simulink model "VehCtrlMdel241025_2018b_amkspdlimit"  (R2019b)
settings: Solver=FixedStepDiscrete  StartTime=0.0  StopTime=30  FixedStep=0.0005  RelTol=1e-3  EnableMultiTasking=on
values from neighbouring files (symbols this model uses):
  Ldwf = 0.4    [VxSpdEstiPara.m]
  Ldwr = 0.5    [VxSpdEstiPara.m]
  thr1 = 0.5    [VxSpdEstiPara.m]
  thr2 = 0.5    [VxSpdEstiPara.m]
  thr3 = 0.5    [VxSpdEstiPara.m]
  thr4 = 0.5    [VxSpdEstiPara.m]
  TrqRquRate = 20    [VxSpdEstiPara.m]
undefined symbols (not defined in the file or in its folder): Ax_OffSet, Ay_OffSet, Caf, Car, DiscIntNeverNeededParam, dwf, dwr, h, i1, i2, I_AN06_5V, I_AN07_5V, I_AN08_5V, I_AN09_5V, I_AN10_5V, I_SW01_L, I_SW02_L, I_SW03_L, I_SW05_L, I_SW07_L, Iz, Kc, Ki, Kp, lf, lr, m, O_SW01_LS0A4, O_SW02_LS0A4, O_SW04_LS0A4, O_SW05_LS0A4, O_SW06_LS0A4, O_SW07_LS0A4, O_SW08_LS0A4, O_SW09_LS0A4, O_SW12_HS1A, O_SW13_HS1A, O_SW14_HS1A, O_SW15_HS1A, Offset_Angle, PWM3, Qa, Ra, RearRatio, Rt, thr5, YawRate_OffSet
libraries: simulink x159, ec5744lib x142, canmsglib x18, MyDesignedModel x1
(part 4 of 6)

== system VehCtrlMdel241025_2018b_amkspdlimit/Input_Processing/Function-Call Subsystem/SWAS ==
  SWAS : Inport
  1-D Lookup Table : Lookup_n-D  NumberOfTableDimensions=1  BreakpointsForDimension1=|  Table=|  InternalRulePriority=Speed  RndMeth=Simplest  InputSameDT=on
      BreakpointsForDimension1=|
      | single([-119.993
      | -109.997
      | -100
      | -90.0034
      | -80.0067
      | -69.9933
      | -59.9966
      | -50
      | -40.0034
      | -30.0067
      | -19.9933
      | -9.99664
      | 0
      | 9.99664
      | 19.9933
      | 30.0067
      | 40.0034
      | 50
      | 59.9966
      | 69.9933
      | 80.0067
      | 90.0034
      | 100
      | 109.997
      | ]);
      Table=|
      | single([-26.072928
      | -23.62248
      | -20.834568
      | -18.002448
      | -15.197904
      | -12.620232
      | -10.131048
      | -8.139672
      | -6.2976672
      | -4.605012
      | -3.0893688
      | -1.4907528
      | -0.07467624
      | 1.40778
      | 2.9621448
      | 4.7211768
      | 6.5521152
      | 8.737056
      | 10.944144
      | 13.743144
      | 17.25012
      | 20.375424
      | 24.070536
      | 27.505584
      | ]);
  1-D Lookup Table1 : Lookup_n-D  NumberOfTableDimensions=1  BreakpointsForDimension1=|  Table=|  InternalRulePriority=Speed  RndMeth=Simplest  InputSameDT=on
      BreakpointsForDimension1=|
      | single([-119.995
      | -109.993
      | -99.9916
      | -90.0067
      | -80.005
      | -70.0034
      | -60.0017
      | -50
      | -39.9983
      | -29.9966
      | -19.995
      | -9.99328
      | 0.00840477
      | 9.99328
      | 19.995
      | 29.9966
      | 39.9983
      | 50
      | 60.0017
      | 70.0034
      | 80.005
      | 90.0067
      | 100.008
      | 109.993
      | ]);
      Table=|
      | single([-26.816256
      | -23.524848
      | -19.851048
      | -16.282584
      | -13.40676
      | -10.314792
      | -7.65504
      | -5.3554968
      | -3.4548912
      | -1.5044184
      | 0.02493504
      | 1.4379192
      | 2.8675296
      | 4.2638976
      | 5.76
      | 7.35588
      | 9.101304
      | 11.04624
      | 12.94128
      | 15.35724
      | 18.244152
      | 20.937168
      | 23.630112
      | 26.306496
      | ]);
  Abs : Abs
  Add1 : Sum
  Add2 : Sum
  Bus Selector : BusSelector  OutputSignals=StrWhlAng,StrWhlAngV
  Bus Creator : BusCreator  Inputs=5
  Cast To Boolean : DataTypeConversion  OutDataTypeStr=single
  Cast To Boolean1 : DataTypeConversion  OutDataTypeStr=single
  Compare To Constant : simulink/Logic and Bit Operations/Compare To Constant  relop=>  const=120  OutDataTypeStr=boolean
  Constant1 : Constant  Value=single(1200)
  Constant2 : Constant  Value=single(1200)
  Constant3 : Constant  Value=single(-1200)
  Constant4 : Constant  Value=single(-1200)
  Constant5 : Constant  Value=single(0.11)
  Gain : Gain  Gain=0.7
  Gain1 : Gain  Gain=0.3
  Gain2 : Gain  Gain=0.7
  Gain3 : Gain  Gain=0.3
  NOT : Logic  Operator=NOT  AllPortsSameDT=off  OutDataTypeStr=boolean
  Rate Limiter Dynamic : simulink/Discontinuities/Rate Limiter Dynamic
      settings: SourceProductName=Simulink
  Rate Limiter Dynamic1 : simulink/Discontinuities/Rate Limiter Dynamic
      settings: SourceProductName=Simulink
  Saturation1 : Saturate  UpperLimit=1200  LowerLimit=0
  Timer : Stateflow chart  TreatAsAtomicUnit=on
  Unit Delay : UnitDelay  SampleTime=-1  HasFrameUpgradeWarning=on
  Unit Delay1 : UnitDelay  SampleTime=-1  HasFrameUpgradeWarning=on
  StrWhlAng&V : Outport  VectorParamsAs1DForOutWhenUnconnected=off
  wires:
  SWAS/1 -> Bus Selector/1
  Bus Selector/2 -> Cast To Boolean1/1  "<StrWhlAngV>"
  Constant3/1 -> Rate Limiter Dynamic/3
  Constant2/1 -> Rate Limiter Dynamic/1
  Gain/1 -> Add2/1
  Gain1/1 -> Add2/2
  Rate Limiter Dynamic/1 -> Abs/1, Gain/1, Unit Delay/1
  Unit Delay/1 -> Gain1/1
  Add2/1 -> 1-D Lookup Table1/1, Bus Creator/4, 1-D Lookup Table/1  "StrWhlAng"
  Bus Creator/1 -> StrWhlAng&V/1
  Add1/1 -> Bus Creator/5  "StrWhlAngV"
  Rate Limiter Dynamic1/1 -> Saturation1/1
  Bus Selector/1 -> Cast To Boolean/1  "<StrWhlAng>"
  Constant1/1 -> Rate Limiter Dynamic1/1
  Constant4/1 -> Rate Limiter Dynamic1/3
  1-D Lookup Table/1 -> Bus Creator/2  "FLWhlStrAng"
  1-D Lookup Table1/1 -> Bus Creator/3  "FRWhlStrAng"
  Unit Delay1/1 -> Gain3/1
  Gain3/1 -> Add1/2
  Gain2/1 -> Add1/1
  Saturation1/1 -> Unit Delay1/1, Gain2/1  "StrWhlAngV"
  Abs/1 -> Compare To Constant/1
  NOT/1 -> Bus Creator/1  "WhlStrAng_Valid"
  Constant5/1 -> Timer/2(CountTime)
  Compare To Constant/1 -> Timer/1(Trigger)  "WhlStrAng_Valid"
  Timer/1(Exit) -> NOT/1
  Cast To Boolean/1 -> Rate Limiter Dynamic/2
  Cast To Boolean1/1 -> Rate Limiter Dynamic1/2

== system VehCtrlMdel241025_2018b_amkspdlimit/Input_Processing/Function-Call Subsystem/Subsystem ==
  note: AMK电机功率计算
  In1 : Inport
  In2 : Inport  Port=2
  In3 : Inport  Port=3
  Bus Selector : BusSelector  OutputSignals=MCFL_ActualTorque,MCFL_ActualVelocity,MCFL_DCVoltage
  Bus Selector1 : BusSelector  OutputSignals=MCFR_ActualTorque,MCFR_ActualVelocity,MCFR_DCVoltage
  Bus Selector2 : BusSelector  OutputSignals=voltage,current
  Constant : Constant  Value=single(9550)
  Constant1 : Constant  Value=single(9550)
  Constant2 : Constant  Value=single(0.01)
  Constant3 : Constant  Value=single(0.01)
  Constant4 : Constant  Value=single(0)
  Constant6 : Constant  Value=single(0)
  Divide{,1..3} (4 alike) : Product  Inputs=*/
  Max : MinMax  Function=max  Inputs=2
  Max1 : MinMax  Function=max  Inputs=2
  MeaModule : ec5744lib/RapidECU_U3/07Calibration/MeaModule  signal=AMKFL_Current
      settings: SourceProductName=ECUCoder for MPC5744
  MeaModule1 : ec5744lib/RapidECU_U3/07Calibration/MeaModule  signal=AMKFR_Current
      settings: SourceProductName=ECUCoder for MPC5744
  MeaModule2 : ec5744lib/RapidECU_U3/07Calibration/MeaModule  signal=EmraxPwr
      settings: SourceProductName=ECUCoder for MPC5744
  Product : Product
  Product1 : Product
  Product2 : Product
  Switch : Switch  Criteria=u2 ~= 0
  Switch1 : Switch  Criteria=u2 ~= 0
  Out1 : Outport
  Out2 : Outport  Port=2
  Out3 : Outport  Port=3
  wires:
  In1/1 -> Bus Selector/1
  In2/1 -> Bus Selector1/1
  Bus Selector/1 -> Product/1  "<MCFL_ActualTorque>"
  Bus Selector/2 -> Product/2  "<MCFL_ActualVelocity>"
  Bus Selector/3 -> Switch/2, Max/1  "<MCFL_DCVoltage>"
  Product/1 -> Divide/1
  Constant/1 -> Divide/2
  Switch/1 -> MeaModule/1  "AMKFL_Current"
  Constant1/1 -> Divide2/2
  Product1/1 -> Divide2/1
  Bus Selector1/3 -> Switch1/2, Max1/1  "<MCFR_DCVoltage>"
  Bus Selector1/1 -> Product1/1  "<MCFR_ActualTorque>"
  Bus Selector1/2 -> Product1/2  "<MCFR_ActualVelocity>"
  Switch1/1 -> MeaModule1/1  "AMKFR_Current"
  MeaModule/1 -> Out1/1
  MeaModule1/1 -> Out2/1
  Constant2/1 -> Max/2
  Max/1 -> Divide1/2
  Constant3/1 -> Max1/2
  Max1/1 -> Divide3/2
  Divide1/1 -> Switch/1  "AMKFL_Current"
  Constant4/1 -> Switch/3
  Constant6/1 -> Switch1/3
  Divide3/1 -> Switch1/1  "AMKFR_Current"
  In3/1 -> Bus Selector2/1
  Bus Selector2/2 -> Product2/2  "<current>"
  Bus Selector2/1 -> Product2/1  "<voltage>"
  Product2/1 -> MeaModule2/1
  MeaModule2/1 -> Out3/1
  Divide/1 -> Divide1/1
  Divide2/1 -> Divide3/1

== system VehCtrlMdel241025_2018b_amkspdlimit/Input_Processing/Function-Call Subsystem/Subsystem1 ==
  In1 : Inport
  Bus Selector : BusSelector  OutputSignals=FLAMKMCUtoVCU1.MCFL_bError,FRAMKMCUtoVCU1.MCFR_bError
  Chart : Stateflow chart  BlockKeywords=__PRM__SERIALIZED__DATA__:Stateflow Chart,Stateflow Diagram  TreatAsAtomicUnit=on
  Constant1 : Constant  Value=single(0.2)
  Detect Rise Positive1 : simulink/Logic and Bit Operations/Detect Rise Positive  vinit=0  OutDataTypeStr=boolean
  OR : Logic  Operator=OR  AllPortsSameDT=off  OutDataTypeStr=boolean
  Timer : Stateflow chart  TreatAsAtomicUnit=on
  AMKerrorTrq_CUT : Outport
  wires:
  In1/1 -> Bus Selector/1
  Bus Selector/1 -> OR/1  "<MCFL_bError>"
  Bus Selector/2 -> OR/2  "<MCFR_bError>"
  OR/1 -> Timer/1(Trigger)
  Constant1/1 -> Timer/2(CountTime)
  Timer/1(Exit) -> Detect Rise Positive1/1
  Detect Rise Positive1/1 -> Chart/1(out1)  "out1"
  Chart/1(Trq_CUT) -> AMKerrorTrq_CUT/1

== system VehCtrlMdel241025_2018b_amkspdlimit/Input_Processing/Function-Call Subsystem/WhlSpdii_mps ==
  IMU : Inport
  In2 : Inport  Port=2
  Bus Selector : BusSelector  OutputSignals=ABS_WS_RL,ABS_WS_RR
  Bus Selector1 : BusSelector  OutputSignals=FRAMKMCUtoVCU1.MCFR_ActualVelocity,FLAMKMCUtoVCU1.MCFL_ActualVelocity
  Bus Creator : BusCreator  Inputs=8
  Compare To Constant{,2,4,6} (4 alike) : simulink/Logic and Bit Operations/Compare To Constant  relop=>=  const=0  OutDataTypeStr=boolean
  Compare To Constant{1,3,5,7} (4 alike) : simulink/Logic and Bit Operations/Compare To Constant  relop=<  const=40  OutDataTypeStr=boolean
  Constant{1,4..5,8} (4 alike) : Constant  Value=single(0.11)
  Constant{2,6,10,12} (4 alike) : Constant  Value=single(10)
  Constant{3,7,11,13} (4 alike) : Constant  Value=single(-10)
  Gain : Gain  Gain=1/3.6
  Gain1 : Gain  Gain=0.4826*3.14/11.3/60
  Gain2 : Gain  Gain=0.4826*3.14/11.3/60
  Gain3 : Gain  Gain=1/3.6
  OR{,1..3} (4 alike) : Logic  Operator=OR  AllPortsSameDT=off  OutDataTypeStr=boolean
  Rate Limiter Dynamic{,1..3} (4 alike) : simulink/Discontinuities/Rate Limiter Dynamic
      settings: SourceProductName=Simulink
  Saturation{,1..3} (4 alike) : Saturate  UpperLimit=30  LowerLimit=0
  Timer : Stateflow chart  TreatAsAtomicUnit=on
  Timer1 : Stateflow chart  TreatAsAtomicUnit=on
  Timer2 : Stateflow chart  TreatAsAtomicUnit=on
  Timer3 : Stateflow chart  TreatAsAtomicUnit=on
  WhlSpdii_mps : Outport  VectorParamsAs1DForOutWhenUnconnected=off
  wires:
  IMU/1 -> Bus Selector/1
  Bus Selector/1 -> Rate Limiter Dynamic/2  "<ABS_WS_RL>"
  Bus Selector/2 -> Rate Limiter Dynamic1/2  "<ABS_WS_RR>"
  Constant2/1 -> Rate Limiter Dynamic/1
  Constant3/1 -> Rate Limiter Dynamic/3
  Constant7/1 -> Rate Limiter Dynamic1/3
  Constant6/1 -> Rate Limiter Dynamic1/1
  Constant10/1 -> Rate Limiter Dynamic2/1
  Constant11/1 -> Rate Limiter Dynamic2/3
  Bus Selector1/1 -> Rate Limiter Dynamic2/2  "<MCFR_ActualVelocity>"
  Bus Selector1/2 -> Rate Limiter Dynamic3/2  "<MCFL_ActualVelocity>"
  Constant13/1 -> Rate Limiter Dynamic3/3
  Constant12/1 -> Rate Limiter Dynamic3/1
  In2/1 -> Bus Selector1/1
  Rate Limiter Dynamic/1 -> Saturation/1
  Rate Limiter Dynamic1/1 -> Saturation1/1
  Rate Limiter Dynamic2/1 -> Saturation2/1
  Rate Limiter Dynamic3/1 -> Saturation3/1
  Saturation/1 -> Gain/1  "WhlSpdRL"
  Saturation1/1 -> Gain3/1  "WhlSpdRR"
  Saturation2/1 -> Gain1/1  "WhlSpdFR"
  Saturation3/1 -> Gain2/1  "WhlSpdFL"
  Bus Creator/1 -> WhlSpdii_mps/1
  Gain2/1 -> Compare To Constant6/1, Compare To Constant7/1, Bus Creator/8  "WhlSpdFL"
  Gain1/1 -> Compare To Constant5/1, Compare To Constant4/1, Bus Creator/6  "WhlSpdFR"
  Gain/1 -> Compare To Constant/1, Compare To Constant1/1, Bus Creator/2  "WhlSpdRL_mps"
  Gain3/1 -> Compare To Constant2/1, Compare To Constant3/1, Bus Creator/4  "WhlSpdRR_mps"
  Compare To Constant/1 -> OR/1
  Compare To Constant1/1 -> OR/2
  Compare To Constant3/1 -> OR1/2
  Compare To Constant2/1 -> OR1/1
  Compare To Constant4/1 -> OR2/1
  Compare To Constant5/1 -> OR2/2
  Compare To Constant7/1 -> OR3/2
  Compare To Constant6/1 -> OR3/1
  Timer/1(Exit) -> Bus Creator/1  "WhlSpdRL_Valid"
  Timer1/1(Exit) -> Bus Creator/3  "WhlSpdRR_Valid"
  Timer2/1(Exit) -> Bus Creator/5  "WhlSpdFR_Valid"
  Timer3/1(Exit) -> Bus Creator/7  "WhlSpdFL_Valid"
  Constant5/1 -> Timer/2(CountTime)
  OR/1 -> Timer/1(Trigger)  "WhlSpdRL_Valid"
  OR1/1 -> Timer1/1(Trigger)  "WhlSpdRR_Valid"
  Constant1/1 -> Timer1/2(CountTime)
  Constant4/1 -> Timer2/2(CountTime)
  OR2/1 -> Timer2/1(Trigger)  "WhlSpdFR_Valid"
  Constant8/1 -> Timer3/2(CountTime)
  OR3/1 -> Timer3/1(Trigger)  "WhlSpdFL_Valid"

== system VehCtrlMdel241025_2018b_amkspdlimit/Input_Processing/Subsystem/IntglJudgment  ==
  note: 对加速度进行积分
  note: 计时器，当积分速度大于轮速一个时间后，退出积分速度。
  note: 积分开始时，需要给初始值
  WhlSlipFL_flag : Inport
  WhlSlipFR_flag : Inport  Port=2
  WhlSlipRL_flag : Inport  Port=3
  WhlSlipRR_flag : Inport  Port=4
  Ax_Valid : Inport  Port=5
  IMU_Ax_mpss : Inport  Port=6
  FFVehVxEst_mps : Inport  Port=7
  Acc_POS : Inport  Port=8
  WhlSpdMax_mps : Inport  Port=9
  AND : Logic  AllPortsSameDT=off  OutDataTypeStr=boolean
  Add{,3..4,10} (4 alike) : Sum
  Add1 : Sum  Inputs=-+
  Add2 : Sum  Inputs=+-
  Cast To Double : DataTypeConversion  OutDataTypeStr=single
  Cast To Double1 : DataTypeConversion  OutDataTypeStr=boolean
  Compare To Constant : simulink/Logic and Bit Operations/Compare To Constant  relop=>  const=TrqRquRate  OutDataTypeStr=boolean
  Compare To Constant1 : simulink/Logic and Bit Operations/Compare To Constant  relop=<=  const=0  OutDataTypeStr=boolean
  Constant : Constant  Value=single(0)
  InitZORE : Constant  Value=single(0)
  Logical Operator : Logic  Operator=OR  Inputs=4  AllPortsSameDT=off  OutDataTypeStr=boolean
  Logical Operator1 : Logic  Operator=NOT  AllPortsSameDT=off  OutDataTypeStr=boolean
  Logical Operator2 : Logic  Operator=OR  AllPortsSameDT=off  OutDataTypeStr=boolean
  Logical Operator3 : Logic  Operator=NOT  AllPortsSameDT=off  OutDataTypeStr=boolean
  Min : MinMax  Inputs=2
  Product : Product
  Relational Operator9 : RelationalOperator  OutDataTypeStr=boolean  RndMeth=Simplest
  Reset : Constant  Value=single(0)
  ResetDelay : Constant  Value=single(0.1)
  Saturation : Saturate  UpperLimit=200  LowerLimit=-10
  Saturation1 : Saturate  UpperLimit=200  LowerLimit=-10
  Steptime : Constant  Value=single(0.01)
  Switch{1,3..4,6} (4 alike) : Switch  Criteria=u2 ~= 0
  Unit Delay{,1..4} (5 alike) : UnitDelay  SampleTime=-1  HasFrameUpgradeWarning=on
  steptime1 : Constant  Value=single(0.01)
  steptime2 : Constant  Value=single(0)
  VxIMU_est : Outport
  IMUVehSpdEstiExit : Outport  Port=2
  wires:
  WhlSlipFL_flag/1 -> Logical Operator/1
  WhlSlipFR_flag/1 -> Logical Operator/2
  WhlSlipRL_flag/1 -> Logical Operator/3
  WhlSlipRR_flag/1 -> Logical Operator/4
  Logical Operator/1 -> Logical Operator1/1
  Unit Delay/1 -> Saturation1/1
  Add/1 -> Switch1/1
  Constant/1 -> Switch1/3
  Logical Operator1/1 -> Logical Operator2/1
  Acc_POS/1 -> Cast To Double/1
  Unit Delay4/1 -> Add1/1
  Add1/1 -> Compare To Constant/1
  Compare To Constant/1 -> Logical Operator2/2
  [IMUAccIns_ACT] -> Switch1/2
  Logical Operator2/1 -> Cast To Double1/1
  Add2/1 -> Compare To Constant1/1
  WhlSpdMax_mps/1 -> Add2/1
  Saturation1/1 -> Add/2
  Product/1 -> Add/1
  IMU_Ax_mpss/1 -> Product/1
  steptime1/1 -> Product/2
  Saturation/1 -> Add3/1
  Add3/1 -> Add2/2, VxIMU_est/1  "VxIMU_est"
  Switch6/1 -> Min/1
  ResetDelay/1 -> Relational Operator9/2, Min/2
  Compare To Constant1/1 -> Switch6/2
  Add10/1 -> Switch6/1
  Steptime/1 -> Add10/2
  Min/1 -> Relational Operator9/1, Unit Delay2/1
  Reset/1 -> Switch6/3
  Unit Delay2/1 -> Add10/1
  Unit Delay3/1 -> Logical Operator3/1
  InitZORE/1 -> Switch4/3
  Logical Operator3/1 -> Switch3/2
  Switch3/1 -> Add3/2, Unit Delay1/1  "VehSpdInit_mps"
  Switch4/1 -> Switch3/1
  Cast To Double/1 -> Unit Delay4/1, Add1/2
  [IMUAccIns_ACT] -> Unit Delay3/1, Switch4/2  "IMUAccIns_ACT"
  Relational Operator9/1 -> IMUVehSpdEstiExit/1  "IMUVehSpdEstiExit"
  Cast To Double1/1 -> AND/2
  Unit Delay1/1 -> Switch3/3
  Add4/1 -> Switch4/1
  FFVehVxEst_mps/1 -> Add4/2
  steptime2/1 -> Add4/1
  Switch1/1 -> Saturation/1, Unit Delay/1
  AND/1 -> [IMUAccIns_ACT]
  Ax_Valid/1 -> AND/1

== system VehCtrlMdel241025_2018b_amkspdlimit/Input_Processing/Subsystem/WhlSlpageJudgment ==
  note: 实践中很难同时满足这三个条件。
      | 一般只满足后两个其中一个即可。
  note: 更改记录：1、理了信号线，更整齐。
      | 2、加速度差，加速度差的微分的判断加入滤波模块。
      | 3、轮速选取改为选取最大轮速。
  note: 选取一个最大轮速
  Vxii_mps : Inport
  IMU_YawRate_dps : Inport  Port=2
  IMU_Aa_mpss : Inport  Port=3
  VehSpdEstiZ1_mps : Inport  Port=4
  In5 : Inport  Port=5
  Bus Selector : BusSelector  OutputSignals=VxFL_mps,VxFR_mps,VxRL_mps,VxRR_mps
  Cast To Double{,1..3} (4 alike) : DataTypeConversion  OutDataTypeStr=boolean
  Constant{1..4} (4 alike) : Constant  Value=single(0.5)
  Logical Operator : Logic  Operator=OR  AllPortsSameDT=off  OutDataTypeStr=boolean
  Logical Operator1 : Logic  AllPortsSameDT=off  OutDataTypeStr=boolean
  Min1 : MinMax  Function=max  Inputs=4
  Mux : Mux
  Mux1 : Mux
  Mux2 : Mux
  Selector : Selector  InputPortWidth=4  IndexOptions=Index vector (dialog)  Indices=[1]  OutputSizes=1
  Selector1 : Selector  InputPortWidth=4  IndexOptions=Index vector (dialog)  Indices=[2]  OutputSizes=1
  Selector2 : Selector  InputPortWidth=4  IndexOptions=Index vector (dialog)  Indices=[3]  OutputSizes=1
  Selector3 : Selector  InputPortWidth=4  IndexOptions=Index vector (dialog)  Indices=[4]  OutputSizes=1
  Terminator : Terminator
  Timer : Stateflow chart  TreatAsAtomicUnit=on
  Timer1 : Stateflow chart  TreatAsAtomicUnit=on
  Timer2 : Stateflow chart  TreatAsAtomicUnit=on
  Timer3 : Stateflow chart  TreatAsAtomicUnit=on
  加速度差判断 : Subsystem
  加速度差的微分的判断 : Subsystem
  速差判断 : Subsystem
  WhlSlipFLValid_flag : Outport
  WhlSlipFRValid_flag : Outport  Port=2
  WhlSlipRLValid_flag : Outport  Port=3
  WhlSlipRRValid_flag : Outport  Port=4
  WhlSpdMax_mps : Outport  Port=5
  wires:
  Selector3/1 -> Cast To Double3/1
  Selector2/1 -> Cast To Double2/1
  [IMU_Aa_mpsss] -> 加速度差的微分的判断/5(IMU_Ax_mpss)
  [VehSpdEstiZ1_mps] -> 速差判断/5(VehSpd_mps)
  Bus Selector/3 -> 加速度差的微分的判断/3(<VxRL_mps>), Min1/3, 速差判断/3(<VxRL_mps>), 加速度差判断/3(<VxRL_mps>)  "<VxRL_mps>"
  Selector1/1 -> Cast To Double1/1
  [IMU_Aa_mpsss] -> 加速度差判断/5(IMU_Ax_mpss)
  Bus Selector/4 -> 加速度差判断/4(<VxRR_mps>), Min1/4, 速差判断/4(<VxRR_mps>), 加速度差的微分的判断/4(<VxRR_mps>)  "<VxRR_mps>"
  IMU_YawRate_dps/1 -> [IMU_YawRate_dps]
  Vxii_mps/1 -> Bus Selector/1
  Bus Selector/1 -> 加速度差的微分的判断/1(<VxFL_mps>), 加速度差判断/1(<VxFL_mps>), Min1/1, 速差判断/1(<VxFL_mps>)  "<VxFL_mps>"
  VehSpdEstiZ1_mps/1 -> [VehSpdEstiZ1_mps]
  Selector/1 -> Cast To Double/1
  Bus Selector/2 -> 加速度差的微分的判断/2(<VxFR_mps>), 加速度差判断/2(<VxFR_mps>), Min1/2, 速差判断/2(<VxFR_mps>)  "<VxFR_mps>"
  IMU_Aa_mpss/1 -> [IMU_Aa_mpsss]
  [IMU_YawRate_dps] -> Terminator/1
  Timer/1(Exit) -> WhlSlipFLValid_flag/1  "WhlSlipFLValid_flag"
  Cast To Double2/1 -> Timer2/1(Trigger)  "WhlSlipRLValid_flag"
  Cast To Double3/1 -> Timer3/1(Trigger)  "WhlSlipRRValid_flag"
  速差判断/1(y) -> Mux/1  "速差"
  速差判断/2(y1) -> Mux/2
  速差判断/3(y2) -> Mux/3
  速差判断/4(y3) -> Mux/4
  加速度差判断/1(y) -> Mux1/1  "加速度差"
  加速度差判断/2(y1) -> Mux1/2
  加速度差判断/3(y2) -> Mux1/3
  加速度差判断/4(y3) -> Mux1/4
  加速度差的微分的判断/1(y) -> Mux2/1  "加速度差的微分"
  加速度差的微分的判断/2(y1) -> Mux2/2
  加速度差的微分的判断/3(y2) -> Mux2/3
  加速度差的微分的判断/4(y3) -> Mux2/4
  Mux1/1 -> Logical Operator/1
  Mux2/1 -> Logical Operator/2
  Mux/1 -> Logical Operator1/1
  Logical Operator/1 -> Logical Operator1/2
  Logical Operator1/1 -> Selector3/1, Selector2/1, Selector1/1, Selector/1
  Min1/1 -> WhlSpdMax_mps/1
  In5/1 -> 速差判断/6(In6)
  Constant1/1 -> Timer/2(CountTime)
  Cast To Double/1 -> Timer/1(Trigger)  "WhlSlipFLValid_flag"
  Timer1/1(Exit) -> WhlSlipFRValid_flag/1  "WhlSlipFRValid_flag"
  Cast To Double1/1 -> Timer1/1(Trigger)  "WhlSlipFRValid_flag"
  Timer2/1(Exit) -> WhlSlipRLValid_flag/1  "WhlSlipRLValid_flag"
  Timer3/1(Exit) -> WhlSlipRRValid_flag/1  "WhlSlipRRValid_flag"
  Constant2/1 -> Timer1/2(CountTime)
  Constant3/1 -> Timer2/2(CountTime)
  Constant4/1 -> Timer3/2(CountTime)

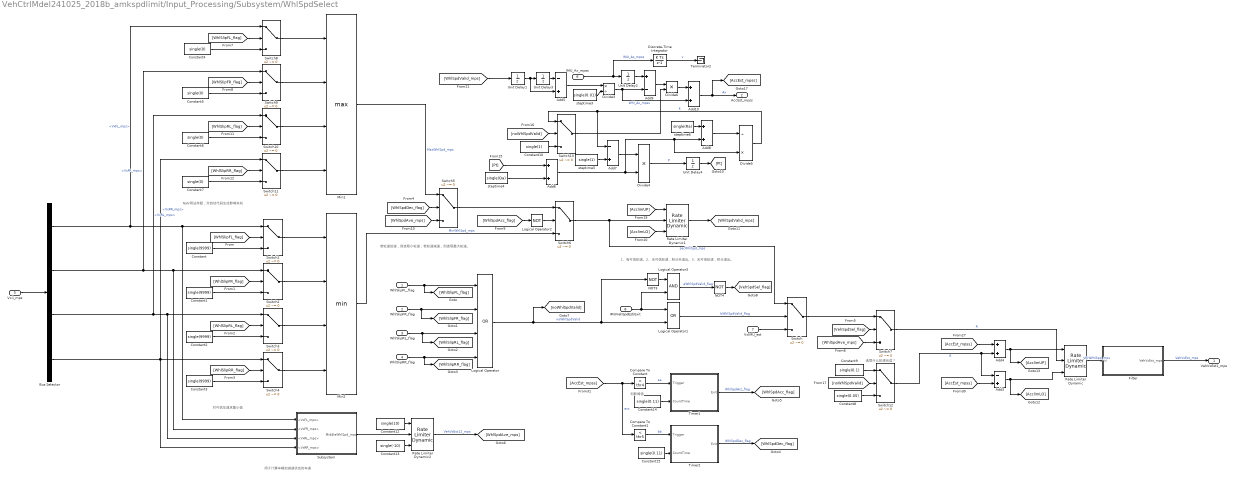
== system VehCtrlMdel241025_2018b_amkspdlimit/Input_Processing/Subsystem/WhlSpdSelect ==
  note: 用于计算车辆加减速状态的车速
  note: 1、有可信轮速。2、无可信轮速，积分未退出。3、无可信轮速，积分退出。
  note: 选取什么轮速合适？
  note: 判断阈值
  note: 若轮速加速，则选取小轮速；若轮速减速，则选取最大轮速。
  note: NaN用法存疑，对自动代码生成影响未知
  note: 对可信车速求最小值
  WhlSlipFL_flag : Inport
  WhlSlipFR_flag : Inport  Port=2
  WhlSlipRL_flag : Inport  Port=3
  WhlSlipRR_flag : Inport  Port=4
  Vxii_mps : Inport  Port=5
  IMU_Ax_mpss : Inport  Port=6
  VxIMU_est : Inport  Port=7
  IMUVehSpdEstiExit : Inport  Port=8
  Add{4,6,8,10} (4 alike) : Sum
  Add3 : Sum  Inputs=-+
  Add5 : Sum  Inputs=-+
  Add7 : Sum  Inputs=-+
  Add9 : Sum  Inputs=+-
  Bus Selector : BusSelector  OutputSignals=VxFL_mps,VxFR_mps,VxRL_mps,VxRR_mps
  Compare To Constant : simulink/Logic and Bit Operations/Compare To Constant  relop=>  const=thr4  OutDataTypeStr=boolean
  Compare To Constant1 : simulink/Logic and Bit Operations/Compare To Constant  relop=<  const=thr5  OutDataTypeStr=boolean
  Constant{,1..3} (4 alike) : Constant  Value=single(9999)
  Constant10 : Constant  Value=single(1)
  Constant12 : Constant  Value=single(10)
  Constant13 : Constant  Value=single(-10)
  Constant14 : Constant  Value=single(0.11)
  Constant15 : Constant  Value=single(0.11)
  Constant{4..7} (4 alike) : Constant  Value=single(0)
  Constant8 : Constant  Value=single(0.05)
  Constant9 : Constant  Value=single(0.1)
  Discrete-Time Integrator : DiscreteIntegrator  SampleTime=-1  ICPrevOutput=DiscIntNeverNeededParam  ICPrevScaledInput=DiscIntNeverNeededParam
  Divide3 : Product  Inputs=*/
  Divide4 : Product  Inputs=**
  Divide5 : Product  Inputs=/*
  Divide6 : Product  Inputs=**
  Filter : Subsystem
  Logical Operator : Logic  Operator=OR  Inputs=4  AllPortsSameDT=off  OutDataTypeStr=boolean
  Logical Operator1 : Logic  Operator=OR  AllPortsSameDT=off  OutDataTypeStr=boolean
  Logical Operator2 : Logic  Operator=NOT  AllPortsSameDT=off  OutDataTypeStr=boolean
  Logical Operator3 : Logic  AllPortsSameDT=off  OutDataTypeStr=boolean
  Min1 : MinMax  Function=max  Inputs=4
  Min2 : MinMax  Inputs=4
  NOT3 : Logic  Operator=NOT  AllPortsSameDT=off  OutDataTypeStr=boolean
  NOT4 : Logic  Operator=NOT  AllPortsSameDT=off  OutDataTypeStr=boolean
  Rate Limiter Dynamic : simulink/Discontinuities/Rate Limiter Dynamic
      settings: SourceProductName=Simulink
  Rate Limiter Dynamic1 : simulink/Discontinuities/Rate Limiter Dynamic
      settings: SourceProductName=Simulink
  Rate Limiter Dynamic2 : simulink/Discontinuities/Rate Limiter Dynamic
      settings: SourceProductName=Simulink
  Subsystem : Subsystem
  Switch{,1..13} (14 alike) : Switch  Criteria=u2 ~= 0
  Terminator2 : Terminator
  Timer1 : Stateflow chart  TreatAsAtomicUnit=on
  Timer2 : Stateflow chart  TreatAsAtomicUnit=on
  Unit Delay1 : UnitDelay  SampleTime=-1  HasFrameUpgradeWarning=on
  Unit Delay2 : UnitDelay  SampleTime=-1  HasFrameUpgradeWarning=on
  Unit Delay3 : UnitDelay  SampleTime=-1  HasFrameUpgradeWarning=on
  Unit Delay4 : UnitDelay  InitialCondition=0.01  SampleTime=-1  HasFrameUpgradeWarning=on
  steptime3 : Constant  Value=single(0.01)
  steptime4 : Constant  Value=single(Qa)
  steptime5 : Constant  Value=single(1)
  steptime6 : Constant  Value=single(Ra)
  VehVxEst1_mps : Outport
  AccEst_mpss : Outport  Port=2
  wires:
  Compare To Constant/1 -> Timer1/1(Trigger)  "aa"
  Vxii_mps/1 -> Bus Selector/1
  WhlSlipRR_flag/1 -> [WhlSlipRR_flag], Logical Operator/4
  Logical Operator3/1 -> NOT4/1  "aWhlSpdValid_flag"
  [VehSpdSel_flag] -> Switch7/2
  Logical Operator2/1 -> Switch6/2
  [WhlSlipFL_flag] -> Switch1/2
  Switch5/1 -> Switch6/1
  Constant/1 -> Switch1/3
  Compare To Constant1/1 -> Timer2/1(Trigger)  "bb"
  [WhlSpdAve_mps] -> Switch5/3
  Constant3/1 -> Switch4/3
  Logical Operator1/1 -> Switch/2  "bWhlSpdValid_flag"
  Switch4/1 -> Min2/4
  Constant2/1 -> Switch3/3
  [WhlSlipRR_flag] -> Switch4/2
  Switch1/1 -> Min2/1
  WhlSlipFR_flag/1 -> [WhlSlipFR_flag], Logical Operator/2
  [WhlSpdAcc_flag] -> Logical Operator2/1
  [WhlSlipRL_flag] -> Switch3/2
  Switch2/1 -> Min2/2
  WhlSlipFL_flag/1 -> [WhlSlipFL_flag], Logical Operator/1
  Constant1/1 -> Switch2/3
  [WhlSpdDec_flag] -> Switch5/2
  [WhlSlipFR_flag] -> Switch2/2
  WhlSlipRL_flag/1 -> [WhlSlipRL_flag], Logical Operator/3
  Switch3/1 -> Min2/3
  [WhlSpdAve_mps] -> Switch7/3
  Bus Selector/1 -> Switch8/1, Subsystem/1(<VxFL_mps>), Switch1/1  "<VxFL_mps>"
  Bus Selector/4 -> Subsystem/4(<VxRR_mps>), Switch11/1, Switch4/1  "<VxRR_mps>"
  [WhlSlipFR_flag] -> Switch9/2
  Bus Selector/2 -> Switch9/1, Subsystem/2(<VxFR_mps>), Switch2/1  "<VxFR_mps>"
  Constant5/1 -> Switch9/3
  Bus Selector/3 -> Switch10/1, Subsystem/3(<VxRL_mps>), Switch3/1  "<VxRL_mps>"
  [WhlSlipRL_flag] -> Switch10/2
  [WhlSlipRR_flag] -> Switch11/2
  Constant6/1 -> Switch10/3
  Constant7/1 -> Switch11/3
  Constant4/1 -> Switch8/3
  [WhlSlipFL_flag] -> Switch8/2
  Switch8/1 -> Min1/1
  Switch9/1 -> Min1/2
  Switch10/1 -> Min1/3
  Switch11/1 -> Min1/4
  Min1/1 -> Switch5/1  "MaxWhlSpd_mps"
  Subsystem/1(MiddleWhlSpd_mps) -> Rate Limiter Dynamic2/2
  Constant12/1 -> Rate Limiter Dynamic2/1
  Constant13/1 -> Rate Limiter Dynamic2/3
  Rate Limiter Dynamic2/1 -> [WhlSpdAve_mps]  "VehVxEst12_mps"
  Min2/1 -> Switch6/3  "MinWhlSpd_mps"
  IMUVehSpdEstiExit/1 -> Logical Operator3/2, Logical Operator1/1
  NOT3/1 -> Logical Operator3/1
  NOT4/1 -> [VehSpdSel_flag]
  Divide5/1 -> Add7/1, Switch13/1  "K"
  Unit Delay3/1 -> Add5/1
  steptime3/1 -> Divide3/2
  Add5/1 -> Divide3/1
  Unit Delay4/1 -> [Pt]
  [Pt] -> Add6/1
  steptime4/1 -> Add6/2
  Add6/1 -> Divide5/2, Add8/2, Divide4/2
  steptime5/1 -> Add7/2
  Add7/1 -> Divide4/1
  Divide4/1 -> Unit Delay4/1  "P"
  steptime6/1 -> Add8/1
  Add8/1 -> Divide5/1
  Divide3/1 -> Add10/2, Add9/2  "Whl_Ax_mpss"
  Add9/1 -> Divide6/1
  Divide6/1 -> Add10/1
  Add10/1 -> AccEst_mpss/1, [AccEst_mpss]  "Ax"
  IMU_Ax_mpss/1 -> Unit Delay2/1, Discrete-Time Integrator/1  "IMU_Ax_mpss"
  VxIMU_est/1 -> Switch/3
  Filter/1(VehVxEst_mps) -> VehVxEst1_mps/1  "VehVxEst_mps"
  Switch/1 -> Switch7/1
  Discrete-Time Integrator/1 -> Terminator2/1  "v"
  [AccEst_mpss] -> Add4/1
  [AccEst_mpss] -> Add3/2
  [WhlSpdValid_mps] -> Unit Delay1/1
  Unit Delay2/1 -> Add9/1
  Switch6/1 -> Switch/1, Rate Limiter Dynamic1/2  "secWhlSpd_mps"
  Add4/1 -> [AcclimUP], Rate Limiter Dynamic/1
  Add3/1 -> [AcclimLO], Rate Limiter Dynamic/3
  Switch7/1 -> Rate Limiter Dynamic/2  "R"
  Rate Limiter Dynamic/1 -> Filter/1(In)  "VEHWhlSpd_mps"
  Rate Limiter Dynamic1/1 -> [WhlSpdValid_mps]
  Unit Delay1/1 -> Add5/2, Unit Delay3/1
  [noWhlSpdValid] -> Switch12/2
  Constant8/1 -> Switch12/3
  Constant9/1 -> Switch12/1
  Switch12/1 -> Add3/1, Add4/2  "R"
  Switch13/1 -> Divide6/2
  [noWhlSpdValid] -> Switch13/2
  Constant10/1 -> Switch13/3
  [AcclimUP] -> Rate Limiter Dynamic1/1
  [AcclimLO] -> Rate Limiter Dynamic1/3
  Logical Operator/1 -> NOT3/1, Logical Operator1/2, [noWhlSpdValid]  "noWhlSpdValid"
  Timer1/1(Exit) -> [WhlSpdAcc_flag]  "WhlSpdAcc_flag"
  Constant14/1 -> Timer1/2(CountTime)
  Timer2/1(Exit) -> [WhlSpdDec_flag]  "WhlSpdDec_flag"
  Constant15/1 -> Timer2/2(CountTime)
  [AccEst_mpss] -> Compare To Constant1/1, Compare To Constant/1  "acc"

== system VehCtrlMdel241025_2018b_amkspdlimit/Input_Processing/Subsystem/坐标系转换 ==
  note: cos模块的单位是弧度制、
  note: 未考虑漂移工况
  note: 顺时针为正，逆时针为负。
  WhlSpdFL_mps : Inport
  WhlSpdFR_mps : Inport  Port=2
  WhlSpdRL_mps : Inport  Port=3
  WhlSpdRR_mps : Inport  Port=4
  IMU_YawRate_dps : Inport  Port=5
  WhlStrAngL_deg : Inport  Port=6
  WhlStrAngR_deg : Inport  Port=7
  Add : Sum  Inputs=+-
  Add1 : Sum
  Add2 : Sum  Inputs=+-
  Add3 : Sum
  Asin : Trigonometry  Operator=cos
  Asin1 : Trigonometry  Operator=cos
  Bus Creator : BusCreator  Inputs=4
  Constant : Constant  Value=single(Ldwr)
  Constant1 : Constant  Value=single(Ldwf)
  Gain : Gain  Gain=1/2
  Gain1 : Gain  Gain=1/2
  Gain2 : Gain  Gain=pi/180
  Gain3 : Gain  Gain=pi/180
  Gain4 : Gain  Gain=pi/180
  Product{,1..3} (4 alike) : Product
  Vxii_mps : Outport
  IMU_YawRate_dps1 : Outport  Port=2
  wires:
  Constant/1 -> Gain/1
  Gain/1 -> Product/2
  IMU_YawRate_dps/1 -> Gain4/1  "IMU_YawRate_dps"
  WhlSpdRL_mps/1 -> Add/1  "WhlSpdRL_mps"
  WhlSpdRR_mps/1 -> Add1/2  "WhlSpdRR_mps"
  Product/1 -> [Vldwr]
  [Vldwr] -> Add/2, Add1/1
  WhlSpdFL_mps/1 -> Product1/1  "WhlSpdFL_mps"
  WhlSpdFR_mps/1 -> Product2/2  "WhlSpdFR_mps"
  Constant1/1 -> Gain1/1
  Gain1/1 -> Product3/1
  Product3/1 -> [Vldwf]
  Product1/1 -> Add2/1  "1"
  [Vldwf] -> Add2/2, Add3/1  "3"
  Product2/1 -> Add3/2
  Add2/1 -> Bus Creator/1  "VxFL_mps"
  Add/1 -> Bus Creator/3  "VxRL_mps"
  Add3/1 -> Bus Creator/2  "VxFR_mps"
  Add1/1 -> Bus Creator/4  "VxRR_mps"
  Bus Creator/1 -> Vxii_mps/1
  Asin1/1 -> Product2/1
  WhlStrAngR_deg/1 -> Gain3/1  "WhlStrAngR_deg"
  WhlStrAngL_deg/1 -> Gain2/1  "WhlStrAngL_deg"
  Asin/1 -> Product1/2  "a"
  Gain2/1 -> Asin/1
  Gain3/1 -> Asin1/1
  Gain4/1 -> IMU_YawRate_dps1/1, Product/1, Product3/2

== system VehCtrlMdel241025_2018b_amkspdlimit/OUTPUT/Beeper/Enabled Subsystem1 ==
  In1 : Inport
  In2 : Inport  Port=2
  Enable : EnablePort
  Chart : Stateflow chart  BlockKeywords=__PRM__SERIALIZED__DATA__:Stateflow Chart,Stateflow Diagram  TreatAsAtomicUnit=on
  Error_State : Outport
  wires:
  In1/1 -> Chart/2(FL)
  In2/1 -> Chart/1(FR)
  Chart/1(LEDOn) -> Error_State/1

== system VehCtrlMdel241025_2018b_amkspdlimit/OUTPUT/Beeper/Subsystem ==
  Enable : EnablePort
  Chart1 : Stateflow chart  BlockKeywords=__PRM__SERIALIZED__DATA__:Stateflow Chart,Stateflow Diagram  TreatAsAtomicUnit=on
  Out1 : Outport
  wires:
  Chart1/1(led) -> Out1/1

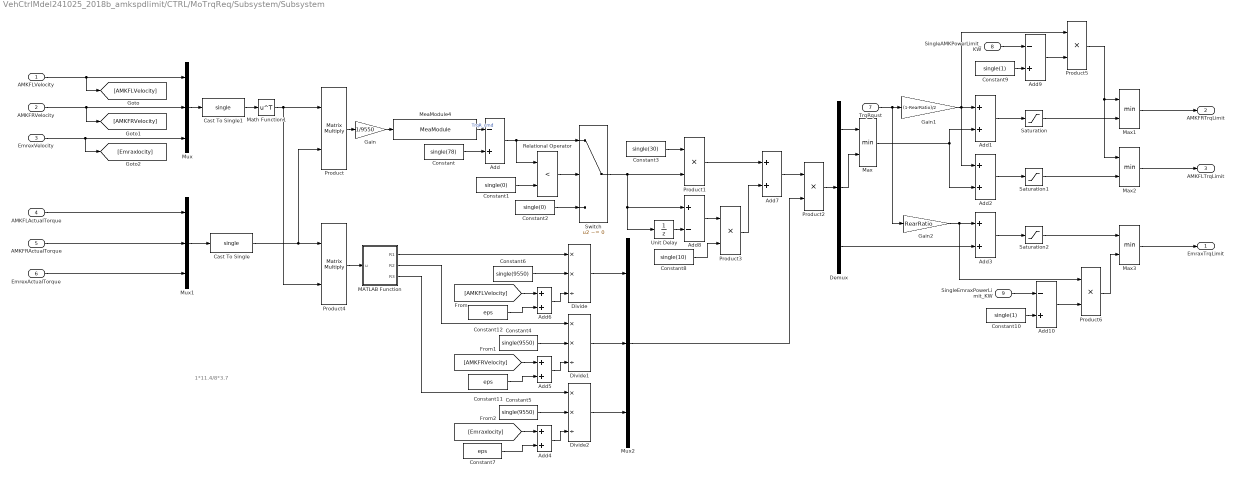
== system VehCtrlMdel241025_2018b_amkspdlimit/CTRL/MoTrqReq/Subsystem/Subsystem ==
  note: 1*11.4/8*3.7
  AMKFLVelocity : Inport
  AMKFRVelocity : Inport  Port=2
  EmrexVelocity : Inport  Port=3
  AMKFLActualTorque : Inport  Port=4
  AMKFRActualTorque : Inport  Port=5
  EmrexActualTorque : Inport  Port=6
  TrqRqust : Inport  Port=7
  SingleAMKPowerLimit_KW : Inport  Port=8
  SingleEmraxPowerLimit_KW : Inport  Port=9
  Add : Sum  Inputs=-+
  Add{1..7} (7 alike) : Sum
  Add10 : Sum  Inputs=-+
  Add8 : Sum  Inputs=+-
  Add9 : Sum  Inputs=-+
  Cast To Single : DataTypeConversion  OutDataTypeStr=single
  Cast To Single1 : DataTypeConversion  OutDataTypeStr=single
  Constant : Constant  Value=single(78)
  Constant1 : Constant  Value=single(0)
  Constant10 : Constant  Value=single(1)
  Constant11 : Constant  Value=eps
  Constant12 : Constant  Value=eps
  Constant2 : Constant  Value=single(0)
  Constant3 : Constant  Value=single(30)
  Constant4 : Constant  Value=single(9550)
  Constant5 : Constant  Value=single(9550)
  Constant6 : Constant  Value=single(9550)
  Constant7 : Constant  Value=eps
  Constant8 : Constant  Value=single(10)
  Constant9 : Constant  Value=single(1)
  Demux : Demux  Outputs=3
  Divide : Product  Inputs=**/
  Divide1 : Product  Inputs=**/
  Divide2 : Product  Inputs=**/
  Gain : Gain  Gain=1/9550
  Gain1 : Gain  Gain=(1-RearRatio)/2
  Gain2 : Gain  Gain=RearRatio
  MATLAB Function : MATLAB Function  TreatAsAtomicUnit=on
  Math Function1 : Math  Operator=transpose  SignedPower=off  SaturateOnIntegerOverflow=on
  Max{,1..3} (4 alike) : MinMax  Inputs=2
  MeaModule4 : ec5744lib/RapidECU_U3/07Calibration/MeaModule  signal=PwrALL
      settings: SourceProductName=ECUCoder for MPC5744
  Mux : Mux  Inputs=3
  Mux1 : Mux  Inputs=3
  Mux2 : Mux  Inputs=3
  Product : Product  Multiplication=Matrix(*)
  Product{1..3,5..6} (5 alike) : Product
  Product4 : Product  Multiplication=Matrix(*)
  Relational Operator : RelationalOperator  Operator=<  OutDataTypeStr=boolean  RndMeth=Simplest
  Saturation : Saturate  UpperLimit=inf  LowerLimit=0
  Saturation1 : Saturate  UpperLimit=inf  LowerLimit=0
  Saturation2 : Saturate  UpperLimit=inf  LowerLimit=0
  Switch : Switch  Criteria=u2 ~= 0
  Unit Delay : UnitDelay  SampleTime=-1  HasFrameUpgradeWarning=on
  EmraxTrqLimit : Outport
  AMKFRTrqLimit : Outport  Port=2
  AMKFLTrqLimit : Outport  Port=3
  wires:
  AMKFLActualTorque/1 -> Mux1/1
  Saturation2/1 -> Max3/1
  MeaModule4/1 -> Add/1  "TrqR_cmd"
  Add1/1 -> Saturation/1
  Math Function1/1 -> Product4/2, Product/1
  EmrexActualTorque/1 -> Mux1/3
  Add8/1 -> Product3/1
  Max/1 -> Add1/2, Add2/2
  Constant5/1 -> Divide2/2
  MATLAB Function/3(R3) -> Divide2/1
  Switch/1 -> Add8/1, Unit Delay/1, Product1/2
  Add3/1 -> Saturation2/1
  Demux/1 -> Max/1
  Constant7/1 -> Add4/2
  SingleAMKPowerLimit_KW/1 -> Add9/1
  Divide2/1 -> Mux2/3
  AMKFRActualTorque/1 -> Mux1/2
  Add6/1 -> Divide/3
  EmrexVelocity/1 -> [Emraxlocity], Mux/3
  MATLAB Function/1(R1) -> Divide/1
  Product4/1 -> MATLAB Function/1(u)
  Cast To Single/1 -> Product4/1, Product/2
  Add/1 -> Switch/1, Relational Operator/1
  TrqRqust/1 -> Gain2/1, Gain1/1
  AMKFLVelocity/1 -> Mux/1, [AMKFLVelocity]
  Constant11/1 -> Add5/2
  Constant4/1 -> Divide1/2
  Gain2/1 -> Product6/1, Add3/1
  Max1/1 -> AMKFRTrqLimit/1
  Divide1/1 -> Mux2/2
  [AMKFRVelocity] -> Add5/1
  Constant2/1 -> Switch/3
  Mux/1 -> Cast To Single1/1
  AMKFRVelocity/1 -> [AMKFRVelocity], Mux/2
  Product6/1 -> Max3/2
  Relational Operator/1 -> Switch/2
  Add4/1 -> Divide2/3
  Product3/1 -> Add7/2
  Product2/1 -> Demux/1
  Add5/1 -> Divide1/3
  MATLAB Function/2(R2) -> Divide1/1
  Constant3/1 -> Product1/1
  Product/1 -> Gain/1
  Mux2/1 -> Product2/2
  Divide/1 -> Mux2/1
  Constant8/1 -> Product3/2
  Add9/1 -> Product5/2
  Demux/3 -> Add3/2
  Constant6/1 -> Divide/2
  Constant/1 -> Add/2
  Gain/1 -> MeaModule4/1
  Product5/1 -> Max2/1, Max1/1
  Constant1/1 -> Relational Operator/2
  Constant12/1 -> Add6/2
  Product1/1 -> Add7/1
  Add7/1 -> Product2/1
  Constant9/1 -> Add9/2
  Gain1/1 -> Product5/1, Add2/1, Add1/1
  Unit Delay/1 -> Add8/2
  SingleEmraxPowerLimit_KW/1 -> Add10/1
  Add10/1 -> Product6/2
  Max3/1 -> EmraxTrqLimit/1
  Saturation/1 -> Max1/2
  Max2/1 -> AMKFLTrqLimit/1
  Add2/1 -> Saturation1/1
  Demux/2 -> Max/2
  Saturation1/1 -> Max2/2
  Cast To Single1/1 -> Math Function1/1
  [AMKFLVelocity] -> Add6/1
  Constant10/1 -> Add10/2
  Mux1/1 -> Cast To Single/1
  [Emraxlocity] -> Add4/1

== system VehCtrlMdel241025_2018b_amkspdlimit/CTRL/MoTrqReq/TCS_PI+FF_Ctrl_FL/Latch_on ==
  Set : Inport
  Reset : Inport  Port=2
  Logical Operator4 : Logic  Operator=NOR  AllPortsSameDT=off  OutDataTypeStr=boolean
  Logical Operator5 : Logic  Operator=NOR  AllPortsSameDT=off  OutDataTypeStr=boolean
  Unit Delay1 : UnitDelay  SampleTime=-1  HasFrameUpgradeWarning=on
  flg_TCSActv : Outport
  wires:
  Logical Operator5/1 -> flg_TCSActv/1, Unit Delay1/1
  Reset/1 -> Logical Operator5/2
  Unit Delay1/1 -> Logical Operator4/1
  Set/1 -> Logical Operator4/2
  Logical Operator4/1 -> Logical Operator5/1

== system VehCtrlMdel241025_2018b_amkspdlimit/CTRL/MoTrqReq/TCS_PI+FF_Ctrl_FL/RisingTimer ==
  Set : Inport
  Timer : Inport  Port=2
  Add10 : Sum
  Min : MinMax  Inputs=2
  Relational Operator9 : RelationalOperator  OutDataTypeStr=boolean  RndMeth=Simplest
  Reset : Constant  Value=single(0)
  Steptime : Constant  Value=single(0.01)
  Switch6 : Switch  Criteria=u2 ~= 0
  Unit Delay1 : UnitDelay  SampleTime=-1  HasFrameUpgradeWarning=on
  TCSExit : Outport
  wires:
  Add10/1 -> Switch6/1
  Set/1 -> Switch6/2
  Min/1 -> Unit Delay1/1, Relational Operator9/1
  Unit Delay1/1 -> Add10/1
  Timer/1 -> Relational Operator9/2, Min/2
  Reset/1 -> Switch6/3
  Relational Operator9/1 -> TCSExit/1
  Steptime/1 -> Add10/2
  Switch6/1 -> Min/1

== system VehCtrlMdel241025_2018b_amkspdlimit/CTRL/MoTrqReq/TCS_PI+FF_Ctrl_FR/Latch_on ==
  Set : Inport
  Reset : Inport  Port=2
  Logical Operator4 : Logic  Operator=NOR  AllPortsSameDT=off  OutDataTypeStr=boolean
  Logical Operator5 : Logic  Operator=NOR  AllPortsSameDT=off  OutDataTypeStr=boolean
  Unit Delay1 : UnitDelay  SampleTime=-1  HasFrameUpgradeWarning=on
  flg_TCSActv : Outport
  wires:
  Logical Operator4/1 -> Logical Operator5/1
  Set/1 -> Logical Operator4/2
  Unit Delay1/1 -> Logical Operator4/1
  Reset/1 -> Logical Operator5/2
  Logical Operator5/1 -> Unit Delay1/1, flg_TCSActv/1

== system VehCtrlMdel241025_2018b_amkspdlimit/CTRL/MoTrqReq/TCS_PI+FF_Ctrl_FR/RisingTimer ==
  Set : Inport
  Timer : Inport  Port=2
  Add10 : Sum
  Min : MinMax  Inputs=2
  Relational Operator9 : RelationalOperator  OutDataTypeStr=boolean  RndMeth=Simplest
  Reset : Constant  Value=single(0)
  Steptime : Constant  Value=single(0.01)
  Switch6 : Switch  Criteria=u2 ~= 0
  Unit Delay1 : UnitDelay  SampleTime=-1  HasFrameUpgradeWarning=on
  TCSExit : Outport
  wires:
  Switch6/1 -> Min/1
  Steptime/1 -> Add10/2
  Relational Operator9/1 -> TCSExit/1
  Reset/1 -> Switch6/3
  Timer/1 -> Min/2, Relational Operator9/2
  Unit Delay1/1 -> Add10/1
  Min/1 -> Relational Operator9/1, Unit Delay1/1
  Set/1 -> Switch6/2
  Add10/1 -> Switch6/1

== system VehCtrlMdel241025_2018b_amkspdlimit/CTRL/MoTrqReq/TCS_PI+FF_Ctrl_R/Latch_on ==
  Set : Inport
  Reset : Inport  Port=2
  Logical Operator4 : Logic  Operator=NOR  AllPortsSameDT=off  OutDataTypeStr=boolean
  Logical Operator5 : Logic  Operator=NOR  AllPortsSameDT=off  OutDataTypeStr=boolean
  Unit Delay1 : UnitDelay  SampleTime=-1  HasFrameUpgradeWarning=on
  flg_TCSActv : Outport
  wires:
  Logical Operator5/1 -> flg_TCSActv/1, Unit Delay1/1
  Reset/1 -> Logical Operator5/2
  Unit Delay1/1 -> Logical Operator4/1
  Set/1 -> Logical Operator4/2
  Logical Operator4/1 -> Logical Operator5/1

== system VehCtrlMdel241025_2018b_amkspdlimit/CTRL/MoTrqReq/TCS_PI+FF_Ctrl_R/RisingTimer ==
  Set : Inport
  Timer : Inport  Port=2
  Add10 : Sum
  Min : MinMax  Inputs=2
  Relational Operator9 : RelationalOperator  OutDataTypeStr=boolean  RndMeth=Simplest
  Reset : Constant  Value=single(0)
  Steptime : Constant  Value=single(0.01)
  Switch6 : Switch  Criteria=u2 ~= 0
  Unit Delay1 : UnitDelay  SampleTime=-1  HasFrameUpgradeWarning=on
  TCSExit : Outport
  wires:
  Add10/1 -> Switch6/1
  Set/1 -> Switch6/2
  Min/1 -> Unit Delay1/1, Relational Operator9/1
  Unit Delay1/1 -> Add10/1
  Timer/1 -> Relational Operator9/2, Min/2
  Reset/1 -> Switch6/3
  Relational Operator9/1 -> TCSExit/1
  Steptime/1 -> Add10/2
  Switch6/1 -> Min/1

== system VehCtrlMdel241025_2018b_amkspdlimit/Input/ABS_Receive/ABS_BUS_state/IMU_state ==
  ID : Inport
  Msg : Inport  Port=2
  Enable : EnablePort
  CAN Unpack1 : canmsglib/CAN Unpack  CANdbFile=d:\Users\YJR\Desktop\DBC\Abs_Dev_Dbc_20240603_NingYuan.dbc  MsgList=(none)  MsgName=ABS_Basic_Msg2  MsgIDType=Standard (11-bit identifier)  MsgIdentifier=1698  MsgLength=8  SignalInfo={'WS_FL','8','16','BE','signed','Standard','0','0.014063','0','-460.8','460.7859';'WS_FR','24','16','BE','signed','Standard','0','0.014063','0','-460.8','460.7859';'WS_RL','40','16','BE','signed','Standard','0','0.014063','0','-460.8','460.7859';'WS_RR','56','16','BE','signed','Standard','0','0.014063','0','-460.8','460.7859'}  IDPort=off  TimestampPort=off  ErrorPort=off  RemotePort=off  LengthPort=off  StatusPort=off  ApplyMinMax=off
      settings: SourceProductName=Simulink Real-Time  SourceProductBaseCode=XP  DataFormat=CANdb specified signals
  CANUnPackMessage4 : ec5744lib/RapidECU_U3/04CANCommunication/CANUnPackMessage  datalength=8  canmessagetype=Standard(11-bit ID)  sampletime=-1
      settings: SourceProductName=ECUCoder for MPC5744
  MeaModule1 : ec5744lib/RapidECU_U3/07Calibration/MeaModule  signal=ABS_WS_FR
      settings: SourceProductName=ECUCoder for MPC5744
  MeaModule2 : ec5744lib/RapidECU_U3/07Calibration/MeaModule  signal=ABS_WS_RL
      settings: SourceProductName=ECUCoder for MPC5744
  MeaModule3 : ec5744lib/RapidECU_U3/07Calibration/MeaModule  signal=ABS_WS_FL
      settings: SourceProductName=ECUCoder for MPC5744
  MeaModule4 : ec5744lib/RapidECU_U3/07Calibration/MeaModule  signal=ABS_WS_RR
      settings: SourceProductName=ECUCoder for MPC5744
  ABS_WS_FR : Outport  VectorParamsAs1DForOutWhenUnconnected=off
  ABS_WS_RL : Outport  Port=2  VectorParamsAs1DForOutWhenUnconnected=off
  ABS_WS_FL : Outport  Port=3  VectorParamsAs1DForOutWhenUnconnected=off
  ABS_WS_RR : Outport  Port=4  VectorParamsAs1DForOutWhenUnconnected=off
  wires:
  CAN Unpack1/3 -> MeaModule2/1  "ABS_WS_RL"
  CAN Unpack1/2 -> MeaModule1/1  "ABS_WS_FR"
  CAN Unpack1/1 -> MeaModule3/1  "ABS_WS_FL"
  CANUnPackMessage4/1 -> CAN Unpack1/1
  ID/1 -> CANUnPackMessage4/1
  Msg/1 -> CANUnPackMessage4/2
  CAN Unpack1/4 -> MeaModule4/1  "ABS_WS_RR"
  MeaModule3/1 -> ABS_WS_FL/1
  MeaModule1/1 -> ABS_WS_FR/1
  MeaModule2/1 -> ABS_WS_RL/1
  MeaModule4/1 -> ABS_WS_RR/1

== system VehCtrlMdel241025_2018b_amkspdlimit/Input/AMKMCU_Receive/FLAMKMCU/AMKMCU_state ==
  CANOK : Inport
  ID : Inport  Port=2
  Msg : Inport  Port=3
  function : TriggerPort  TriggerType=function-call  VariantControl=(inherit)
  MCU_state : Subsystem  TreatAsAtomicUnit=on
  FLAMKtoVCU1 : Outport  VectorParamsAs1DForOutWhenUnconnected=off
  wires:
  Msg/1 -> MCU_state/2(Msg)
  CANOK/1 -> MCU_state/Enable
  ID/1 -> MCU_state/1(ID)
  MCU_state/1(FLAMKMCUtoVCU1) -> FLAMKtoVCU1/1

== system VehCtrlMdel241025_2018b_amkspdlimit/Input/AMKMCU_Receive/FLAMKMCU/AMKMCU_state1 ==
  CANOK : Inport
  ID : Inport  Port=2
  Msg : Inport  Port=3
  function : TriggerPort  TriggerType=function-call  VariantControl=(inherit)
  Bus Creator : BusCreator  Inputs=2
  MCU_state : Subsystem  TreatAsAtomicUnit=on
  FLAMKMCUtoVCU2 : Outport  VectorParamsAs1DForOutWhenUnconnected=off
  wires:
  MCU_state/2(MCFL_ErrorInfo) -> Bus Creator/2
  MCU_state/1(MCFL_DiagnosticNum) -> Bus Creator/1
  Bus Creator/1 -> FLAMKMCUtoVCU2/1
  ID/1 -> MCU_state/1(ID)
  CANOK/1 -> MCU_state/Enable
  Msg/1 -> MCU_state/2(Msg)

== system VehCtrlMdel241025_2018b_amkspdlimit/Input/AMKMCU_Receive/FLAMKMCU/AMKMCU_state2 ==
  CANOK : Inport
  ID : Inport  Port=2
  Msg : Inport  Port=3
  function : TriggerPort  TriggerType=function-call  VariantControl=(inherit)
  Bus Creator : BusCreator  Inputs=3
  MCU_state : Subsystem  TreatAsAtomicUnit=on
  FLAMKMCUtoVCU3 : Outport  VectorParamsAs1DForOutWhenUnconnected=off
  wires:
  Msg/1 -> MCU_state/2(Msg)
  CANOK/1 -> MCU_state/Enable
  ID/1 -> MCU_state/1(ID)
  Bus Creator/1 -> FLAMKMCUtoVCU3/1  "Bus Creator"
  MCU_state/1(MCFL_TempIGBT) -> Bus Creator/1
  MCU_state/2(MCFL_TempInverter) -> Bus Creator/2
  MCU_state/3(MCFL_TempMotor) -> Bus Creator/3

== system VehCtrlMdel241025_2018b_amkspdlimit/Input/AMKMCU_Receive/FRAMKMCU/AMKMCU_state ==
  CANOK : Inport
  ID : Inport  Port=2
  Msg : Inport  Port=3
  function : TriggerPort  TriggerType=function-call  VariantControl=(inherit)
  Bus Creator : BusCreator  Inputs=12
  MCU_state : Subsystem  TreatAsAtomicUnit=on
  FRAMKMCUtoVCU1 : Outport  VectorParamsAs1DForOutWhenUnconnected=off
  wires:
  ID/1 -> MCU_state/1(ID)
  CANOK/1 -> MCU_state/Enable
  Msg/1 -> MCU_state/2(Msg)
  MCU_state/1(MCFR_ActualTorque) -> Bus Creator/1
  MCU_state/2(MCFR_ActualVelocity) -> Bus Creator/2
  MCU_state/3(MCFR_DCVoltage) -> Bus Creator/3
  MCU_state/4(MCFR_bDCOn) -> Bus Creator/4
  MCU_state/5(MCFR_bDerating) -> Bus Creator/5
  MCU_state/6(MCFR_bError) -> Bus Creator/6
  MCU_state/7(MCFR_bInverterOn) -> Bus Creator/7
  MCU_state/8(MCFR_bQuitDCOn) -> Bus Creator/8
  MCU_state/9(MCFR_bQuitInverterOn) -> Bus Creator/9
  MCU_state/10(MCFR_bReserve) -> Bus Creator/10
  MCU_state/11(MCFR_bSystemReady) -> Bus Creator/11
  MCU_state/12(MCFR_bWarn) -> Bus Creator/12
  Bus Creator/1 -> FRAMKMCUtoVCU1/1

== system VehCtrlMdel241025_2018b_amkspdlimit/Input/AMKMCU_Receive/FRAMKMCU/AMKMCU_state1 ==
  CANOK : Inport
  ID : Inport  Port=2
  Msg : Inport  Port=3
  function : TriggerPort  TriggerType=function-call  VariantControl=(inherit)
  Bus Creator : BusCreator  Inputs=2
  MCU_state : Subsystem  TreatAsAtomicUnit=on
  FRAMKMCUtoVCU2 : Outport  VectorParamsAs1DForOutWhenUnconnected=off
  wires:
  Msg/1 -> MCU_state/2(Msg)
  CANOK/1 -> MCU_state/Enable
  ID/1 -> MCU_state/1(ID)
  Bus Creator/1 -> FRAMKMCUtoVCU2/1
  MCU_state/1(MCFR_DiagnosticNum) -> Bus Creator/1
  MCU_state/2(MCFR_ErrorInfo) -> Bus Creator/2

== system VehCtrlMdel241025_2018b_amkspdlimit/Input/AMKMCU_Receive/FRAMKMCU/AMKMCU_state2 ==
  CANOK : Inport
  ID : Inport  Port=2
  Msg : Inport  Port=3
  function : TriggerPort  TriggerType=function-call  VariantControl=(inherit)
  Bus Creator : BusCreator  Inputs=3
  MCU_state : Subsystem  TreatAsAtomicUnit=on
  FRAMKMCUtoVCU3 : Outport  VectorParamsAs1DForOutWhenUnconnected=off
  wires:
  Bus Creator/1 -> FRAMKMCUtoVCU3/1
  ID/1 -> MCU_state/1(ID)
  CANOK/1 -> MCU_state/Enable
  Msg/1 -> MCU_state/2(Msg)
  MCU_state/1(MCFR_TempIGBT) -> Bus Creator/1
  MCU_state/2(MCFR_TempInverter) -> Bus Creator/2
  MCU_state/3(MCFR_TempMotor) -> Bus Creator/3

== system VehCtrlMdel241025_2018b_amkspdlimit/Input/BMS_Recive/ABS_BUS_state/IMU_state ==
  ID : Inport
  Msg : Inport  Port=2
  Enable : EnablePort
  CAN Unpack1 : canmsglib/CAN Unpack  CANdbFile=d:\Users\YJR\Desktop\DBC\bms.dbc  MsgList=(none)  MsgName=BMS_HCU_INFO  MsgIDType=Extended (29-bit identifier)  MsgIdentifier=408961267  MsgLength=8  SignalInfo={'BatAlmlv','52','4','LE','signed','Standard','0','1','0','0','4';'BatLife','56','8','LE','signed','Standard','0','1','0','0','255';'BatState','48','4','LE','signed','Standard','0','1','0','0','7';'LSBAz','24','8','LE','signed','Standard','0','0.1','-1000','-1012.8','-987.3';'LSBVz','8','8','LE','unsigned','Standard','0','0.1','0','0','9000';'MSBAz','16','8','LE','unsigned','Standard','0','0.1','-1000','-1000','-974.5';'MSBVz','0','8','LE','unsigned','Standard','0','0.1','0','0','9000';'SOCz','32','8','LE','signed','Standard','0','1','0','0','100';'SOHz','40','8','LE','signed','Standard','0','1','0','0','100'}  IDPort=off  TimestampPort=off  ErrorPort=off  RemotePort=off  LengthPort=off  StatusPort=off  ApplyMinMax=off
      settings: SourceProductName=Simulink Real-Time  SourceProductBaseCode=XP  DataFormat=CANdb specified signals
  CANUnPackMessage4 : ec5744lib/RapidECU_U3/04CANCommunication/CANUnPackMessage  datalength=8  canmessagetype=Extended(29-bit ID)  sampletime=-1
      settings: SourceProductName=ECUCoder for MPC5744
  BatAlmlv : Outport  VectorParamsAs1DForOutWhenUnconnected=off
  BatLife : Outport  Port=2  VectorParamsAs1DForOutWhenUnconnected=off
  BatState : Outport  Port=3  VectorParamsAs1DForOutWhenUnconnected=off
  LSBAz : Outport  Port=4  VectorParamsAs1DForOutWhenUnconnected=off
  LSBVz : Outport  Port=5  VectorParamsAs1DForOutWhenUnconnected=off
  MSBAz : Outport  Port=6  VectorParamsAs1DForOutWhenUnconnected=off
  MSBVz : Outport  Port=7  VectorParamsAs1DForOutWhenUnconnected=off
  SOCz : Outport  Port=8  VectorParamsAs1DForOutWhenUnconnected=off
  SOHz : Outport  Port=9  VectorParamsAs1DForOutWhenUnconnected=off
  wires:
  CANUnPackMessage4/1 -> CAN Unpack1/1
  ID/1 -> CANUnPackMessage4/1
  Msg/1 -> CANUnPackMessage4/2
  CAN Unpack1/1 -> BatAlmlv/1  "BatAlmlv"
  CAN Unpack1/2 -> BatLife/1  "BatLife"
  CAN Unpack1/3 -> BatState/1  "BatState"
  CAN Unpack1/4 -> LSBAz/1  "LSBAz"
  CAN Unpack1/5 -> LSBVz/1  "LSBVz"
  CAN Unpack1/6 -> MSBAz/1  "MSBAz"
  CAN Unpack1/7 -> MSBVz/1  "MSBVz"
  CAN Unpack1/8 -> SOCz/1  "SOCz"
  CAN Unpack1/9 -> SOHz/1  "SOHz"
